simulink model "Robot_Static2"  (R2025b)
settings: Solver=VariableStepAuto  StartTime=0.0  StopTime=1500  FixedStep=0.01  RelTol=1e-3
undefined symbols (not defined in the file): Brick_x, Brick_y, Brick_z, C_tile_force, C_tile_torque, Container_x, Container_y, Container_z, J_B_B_SIM, J_C_C_SIM, J_P_P_SIM, J_T_T_SIM, K_tile_force, K_tile_torque, m_B_SIM, m_C_SIM, m_P_SIM, m_T_SIM, q_traj, robot, X, Y, Z
libraries: nesl_utility x181, sm_lib x115
(part 9 of 9)

== system Robot_Static2/Subsystem/Tile7/Grab/Force ==
  pos : Inport
  vel : Inport  Port=2
  Constant : Constant  Value=K_tile_force
  Constant1 : Constant  Value=C_tile_force
  Product : Product
  Product1 : Product
  Sum : Sum  Inputs=--
  Mating : Outport
  wires:
  Constant/1 -> Product/1
  Constant1/1 -> Product1/2
  Product/1 -> Sum/1
  Product1/1 -> Sum/2
  Sum/1 -> Mating/1
  pos/1 -> Product/2
  vel/1 -> Product1/1

== system Robot_Static2/Subsystem/Tile7/Grab/Torque ==
  EA : Inport
  Omega : Inport  Port=2
  Constant : Constant  Value=K_tile_torque
  Constant1 : Constant  Value=C_tile_torque
  Product : Product
  Product1 : Product
  Sum : Sum  Inputs=--
  Mating : Outport
  wires:
  Omega/1 -> Product1/1
  EA/1 -> Product/2
  Sum/1 -> Mating/1
  Product1/1 -> Sum/2
  Product/1 -> Sum/1
  Constant1/1 -> Product1/2
  Constant/1 -> Product/1

== system Robot_Static2/Subsystem/Tile7/Starting Position/Force ==
  pos : Inport
  vel : Inport  Port=2
  Constant : Constant  Value=150000
  Constant1 : Constant  Value=8000
  Product : Product
  Product1 : Product
  Sum : Sum  Inputs=--
  Mating Force : Outport
  wires:
  Constant/1 -> Product/1
  Constant1/1 -> Product1/2
  Product/1 -> Sum/1
  Product1/1 -> Sum/2
  Sum/1 -> Mating Force/1
  pos/1 -> Product/2
  vel/1 -> Product1/1

== system Robot_Static2/Subsystem/Tile7/Starting Position/Torque ==
  EA : Inport
  Omega : Inport  Port=2
  Constant : Constant  Value=150000
  Constant1 : Constant  Value=8000
  Product : Product
  Product1 : Product
  Sum : Sum  Inputs=--
  Mating Torque : Outport
  wires:
  Omega/1 -> Product1/1
  EA/1 -> Product/2
  Sum/1 -> Mating Torque/1
  Product1/1 -> Sum/2
  Product/1 -> Sum/1
  Constant1/1 -> Product1/2
  Constant/1 -> Product/1

== stateflow chart Robot_Static2/Subsystem/Tile4/One Tile Strategy ==
  state Start
    Container_Mating = 1;
    Arm_Mating = 0;
    Antenna_Mating = 0;
  state Grabbing___carring
    Container_Mating = 0;
    Arm_Mating = 1;
    Antenna_Mating = 0;
  state Deposing
    Container_Mating = 0;
    Arm_Mating = 0;
    Antenna_Mating = 1;
  (default) -> Start
  Start -> Grabbing___carring : [dist_arm <= 0.015 && EA_arm<=10*pi/180]
  Grabbing___carring -> Deposing : [dist_endpoint <= 0.015 && EA_endpoint<=10*pi/180]
  data: dist_endpoint input; EA_endpoint input; dist_arm input; Arm_Mating output; Container_Mating output; Antenna_Mating output; EA_arm input

== stateflow chart Robot_Static2/Subsystem/Tile5/One Tile Strategy ==
  state Start
    Container_Mating = 1;
    Arm_Mating = 0;
    Antenna_Mating = 0;
  state Grabbing___carring
    Container_Mating = 0;
    Arm_Mating = 1;
    Antenna_Mating = 0;
  state Deposing
    Container_Mating = 0;
    Arm_Mating = 0;
    Antenna_Mating = 1;
  (default) -> Start
  Start -> Grabbing___carring : [dist_arm <= 0.015 && EA_arm<=10*pi/180]
  Grabbing___carring -> Deposing : [dist_endpoint <= 0.015 && EA_endpoint<=10*pi/180]
  data: dist_endpoint input; EA_endpoint input; dist_arm input; Arm_Mating output; Container_Mating output; Antenna_Mating output; EA_arm input

== stateflow chart Robot_Static2/Subsystem/Tile6/One Tile Strategy ==
  state Start
    Container_Mating = 1;
    Arm_Mating = 0;
    Antenna_Mating = 0;
  state Grabbing___carring
    Container_Mating = 0;
    Arm_Mating = 1;
    Antenna_Mating = 0;
  state Deposing
    Container_Mating = 0;
    Arm_Mating = 0;
    Antenna_Mating = 1;
  (default) -> Start
  Start -> Grabbing___carring : [dist_arm <= 0.015 && EA_arm<=10*pi/180]
  Grabbing___carring -> Deposing : [dist_endpoint <= 0.015 && EA_endpoint<=10*pi/180]
  data: dist_endpoint input; EA_endpoint input; dist_arm input; Arm_Mating output; Container_Mating output; Antenna_Mating output; EA_arm input

== stateflow chart Robot_Static2/Subsystem/Tile7/One Tile Strategy ==
  state Start
    Container_Mating = 1;
    Arm_Mating = 0;
    Antenna_Mating = 0;
  state Grabbing___carring
    Container_Mating = 0;
    Arm_Mating = 1;
    Antenna_Mating = 0;
  state Deposing
    Container_Mating = 0;
    Arm_Mating = 0;
    Antenna_Mating = 1;
  (default) -> Start
  Start -> Grabbing___carring : [dist_arm <= 0.015 && EA_arm<=10*pi/180]
  Grabbing___carring -> Deposing : [dist_endpoint <= 0.015 && EA_endpoint<=10*pi/180]
  data: dist_endpoint input; EA_endpoint input; dist_arm input; Arm_Mating output; Container_Mating output; Antenna_Mating output; EA_arm input

== stateflow chart Robot_Static2/Subsystem/Tile1/One Tile Strategy ==
  state Start
    Container_Mating = 1;
    Arm_Mating = 0;
    Antenna_Mating = 0;
  state Grabbing___carring
    Container_Mating = 0;
    Arm_Mating = 1;
    Antenna_Mating = 0;
  state Deposing
    Container_Mating = 0;
    Arm_Mating = 0;
    Antenna_Mating = 1;
  (default) -> Start
  Start -> Grabbing___carring : [dist_arm <= 0.015 && EA_arm<=10*pi/180]
  Grabbing___carring -> Deposing : [dist_endpoint <= 0.015 && EA_endpoint<=10*pi/180]
  data: dist_endpoint input; EA_endpoint input; dist_arm input; Arm_Mating output; Container_Mating output; Antenna_Mating output; EA_arm input

== stateflow chart Robot_Static2/Subsystem/Tile2/One Tile Strategy ==
  state Start
    Container_Mating = 1;
    Arm_Mating = 0;
    Antenna_Mating = 0;
  state Grabbing___carring
    Container_Mating = 0;
    Arm_Mating = 1;
    Antenna_Mating = 0;
  state Deposing
    Container_Mating = 0;
    Arm_Mating = 0;
    Antenna_Mating = 1;
  (default) -> Start
  Start -> Grabbing___carring : [dist_arm <= 0.015 && EA_arm<=10*pi/180]
  Grabbing___carring -> Deposing : [dist_endpoint <= 0.015 && EA_endpoint<=10*pi/180]
  data: dist_endpoint input; EA_endpoint input; dist_arm input; Arm_Mating output; Container_Mating output; Antenna_Mating output; EA_arm input

== stateflow chart Robot_Static2/Subsystem/Tile3/One Tile Strategy ==
  state Start
    Container_Mating = 1;
    Arm_Mating = 0;
    Antenna_Mating = 0;
  state Grabbing___carring
    Container_Mating = 0;
    Arm_Mating = 1;
    Antenna_Mating = 0;
  state Deposing
    Container_Mating = 0;
    Arm_Mating = 0;
    Antenna_Mating = 1;
  (default) -> Start
  Start -> Grabbing___carring : [dist_arm <= 0.015 && EA_arm<=10*pi/180]
  Grabbing___carring -> Deposing : [dist_endpoint <= 0.015 && EA_endpoint<=10*pi/180]
  data: dist_endpoint input; EA_endpoint input; dist_arm input; Arm_Mating output; Container_Mating output; Antenna_Mating output; EA_arm input
